simulink model "EC_control"  (R2023b)
settings: Solver=FixedStepAuto  StartTime=0.0  StopTime=inf  RelTol=1e-4  AbsTol=1e-6
undefined symbols (not defined in the file): Tr_nom_v, Trx_Ratio
libraries: eeGeneralControl x2, simulink x1
settings Model: ModifiedByFormat=Third Equation Ltd  Creator=Third Equation Ltd  LastModifiedBy=Third Equation Ltd
settings SolverCC: AutoScaleAbsTol=off  AlgebraicLoopSolver=TrustRegion  MaxZcPerStep=1
settings DataIOCC: ExternalInput=[]  InitialState=[]  SaveFormat=Array  SaveOutput=off  SaveTime=off  ReturnWorkspaceOutputs=off
settings OptimizationCC: BlockReduction=off  BooleanDataType=off  ReuseModelBlockBuffer=off  ExpressionDepthLimit=2147483647  InitFltsAndDblsToZero=on
settings DebuggingCC: SaveWithParameterizedLinksMsg=none  SignalResolutionControl=TryResolveAllWithWarning  MultiTaskDSMMsg=warning  MultiTaskCondExecSysMsg=none  IntegerOverflowMsg=none  FcnCallInpInsideContextMsg=warning  UnconnectedInputMsg=warning  UnconnectedOutputMsg=warning  UnconnectedLineMsg=warning  StateNameClashWarn=warning  SFUnexpectedBacktrackingDiag=warning  SFNoUnconditionalDefaultTransitionDiag=warning  SFExecutionAtInitializationDiag=none  IntegerSaturationMsg=none  UnderSpecifiedDimensionMsg=warning  ArithmeticOperatorsInVariantConditions=warning
settings HardwareCC: ProdBitPerPointer=32  ProdBitPerSizeT=32  ProdBitPerPtrDiffT=32  ProdLargestAtomicFloat=None  ProdWordSize=32  ProdHWDeviceType=Custom Processor->Custom Processor
settings ModelReferenceCC: EnableRefExpFcnMdlSchedulingChecks=on  PropagateSignalLabelsOutOfModel=off
settings SFSimCC: SimUseLocalCustomCode=off  CustomCodeUndefinedFunction=UseInterfaceOnly
settings RTWCC: Description=FMU2CS  SystemTargetFile=fmu2cs.tlc  TemplateMakefile=fmu2cs_default_tmf  RTWUseLocalCustomCode=off  DLArmComputeVersion=19.05
settings CodeAppCC: StateflowObjectComments=on
settings GRTTargetCC: TargetLangStandard=C89/C90 (ANSI)  CombineOutputUpdateFcns=off  MatFileLogging=off
settings ConfigComp: CovMetricSettings=dw  CovSaveCumulativeToWorkspaceVar=on  CovSaveSingleToWorkspaceVar=on  CovExternalEMLEnable=off  CovSFcnEnable=off

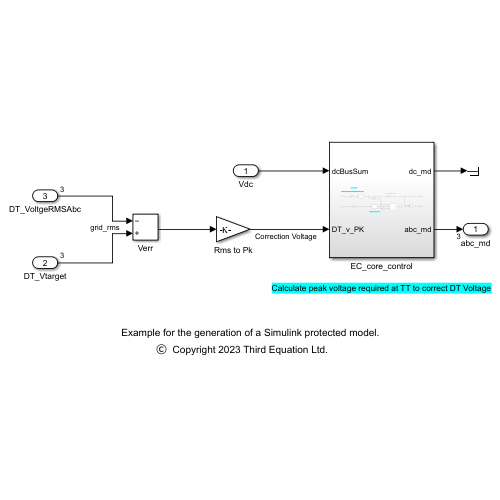
[thumbnail: Simulink's stored preview of the top-level diagram]
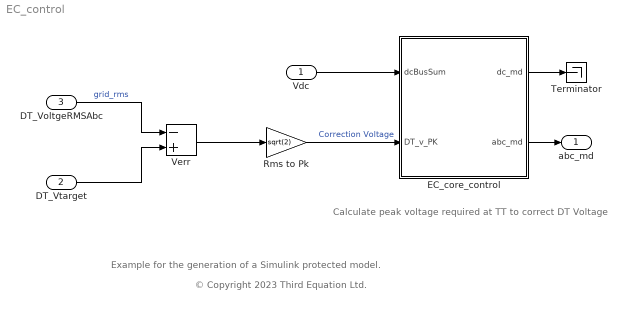
== system EC_control ==
  note: Example for the generation of a Simulink protected model.
  note: © Copyright 2023 Third Equation Ltd.
  note: Calculate peak voltage required at TT to correct DT Voltage
  Vdc : Inport  OutDataTypeStr=single  PortDimensions=1
  DT_Vtarget : Inport  Port=2  OutDataTypeStr=single  Unit=V  PortDimensions=3
  DT_VoltgeRMSAbc : Inport  Port=3  OutDataTypeStr=single  Unit=V  PortDimensions=3
  EC_core_control : Subsystem
  Rms to Pk : Gain  Gain=sqrt(2)  ParamDataTypeStr=single  OutDataTypeStr=single
  Terminator : Terminator
  Verr : Sum  Inputs=-+  OutDataTypeStr=single  AccumDataTypeStr=single
  abc_md : Outport  OutDataTypeStr=single  PortDimensions=3
  wires:
  EC_core_control/1(dc_md) -> Terminator/1
  EC_core_control/2(abc_md) -> abc_md/1
  DT_Vtarget/1 -> Verr/2
  Verr/1 -> Rms to Pk/1
  DT_VoltgeRMSAbc/1 -> Verr/1  "grid_rms"
  Rms to Pk/1 -> EC_core_control/2(DT_v_PK)  "Correction Voltage"
  Vdc/1 -> EC_core_control/1(dcBusSum)

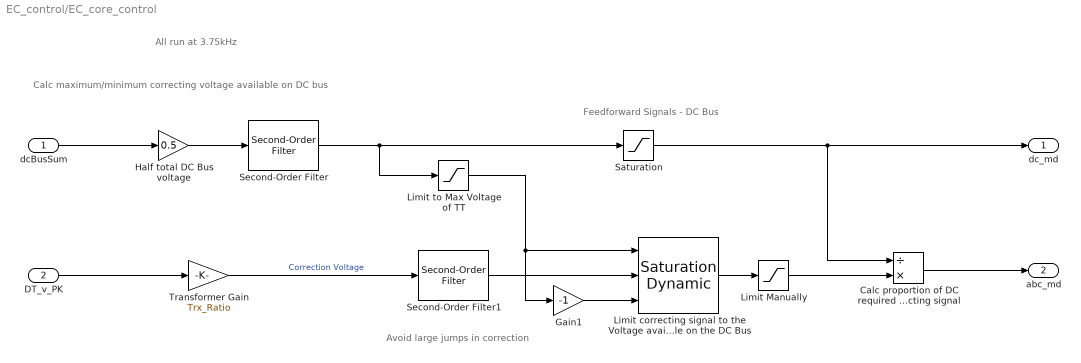
== system EC_control/EC_core_control ==
  note: Avoid large jumps in correction
  note: Calc maximum/minimum correcting voltage available on DC bus
  note: Feedforward Signals - DC Bus
  note: All run at 3.75kHz
  dcBusSum : Inport  OutDataTypeStr=single  Unit=V
  DT_v_PK : Inport  Port=2
  Calc proportion of DC required for correcting signal : Product  Inputs=/*  OutDataTypeStr=single
  Gain1 : Gain  Gain=-1  ParamDataTypeStr=single  OutDataTypeStr=single
  Half total DC Bus voltage : Gain  Gain=0.5  ParamDataTypeStr=single  OutDataTypeStr=single
  Limit Manually : Saturate  UpperLimit=400  LowerLimit=-400  OutDataTypeStr=single
  Limit correcting signal to the Voltage available on the DC Bus : simulink/Discontinuities/Saturation Dynamic  OutMin=[]  OutMax=[]  OutDataTypeStr=single  OutputDataTypeScalingMode=single  OutDataType=fixdt(1, 16)  OutScaling=2^-10  DoSatur=off
  Limit to Max Voltage of TT : Saturate  UpperLimit=Tr_nom_v*sqrt(2)  LowerLimit=0  OutDataTypeStr=single
  Saturation : Saturate  UpperLimit=1000  LowerLimit=50  OutDataTypeStr=single
  Second-Order Filter : eeGeneralControl/Second-Order Filter  FilterType=Low-pass  fn=single(1)  Zeta=single(0.707)  Ts=-1  A0=0  Ph0=0  f0=0  b0=0
  Second-Order Filter1 : eeGeneralControl/Second-Order Filter  FilterType=Low-pass  fn=single(1)  Zeta=single(0.707)  Ts=-1  A0=0  Ph0=0  f0=0  b0=0
  Transformer Gain : Gain  Gain=Trx_Ratio  ParamDataTypeStr=single  OutDataTypeStr=single
  dc_md : Outport
  abc_md : Outport  Port=2
  wires:
  Limit correcting signal to the Voltage available on the DC Bus/1 -> Limit Manually/1
  Saturation/1 -> Calc proportion of DC required for correcting signal/1, dc_md/1
  Limit Manually/1 -> Calc proportion of DC required for correcting signal/2
  dcBusSum/1 -> Half total DC Bus voltage/1
  Second-Order Filter1/1 -> Limit correcting signal to the Voltage available on the DC Bus/2
  Limit to Max Voltage of TT/1 -> Gain1/1, Limit correcting signal to the Voltage available on the DC Bus/1
  Gain1/1 -> Limit correcting signal to the Voltage available on the DC Bus/3
  Second-Order Filter/1 -> Limit to Max Voltage of TT/1, Saturation/1
  Half total DC Bus voltage/1 -> Second-Order Filter/1
  Calc proportion of DC required for correcting signal/1 -> abc_md/1
  Transformer Gain/1 -> Second-Order Filter1/1  "Correction Voltage"
  DT_v_PK/1 -> Transformer Gain/1
